simulink model "C_PTES_sim_v2"  (R2025a)
settings: Solver=ode23tb  StartTime=0.0  StopTime=600
PreLoadFcn:
  | Load_Maps
InitFcn:
  | A_init_compressor
StopFcn:
  | % AB_plotHX
  | % AB_plotmap
model workspace (MAT data in the model file):
  Step_time = 1000
  step_time = 200
values from neighbouring files (symbols this model uses):
  DeltaW = 0    [A_init_compressor.m]    (also in B_init_compressor.m = input('Power change: '))
  Ki_tau = 23.1297    [A_init_compressor.m]    (also in B_init_compressor.m = 0.1)
  Kp_tau = 289.6844    [A_init_compressor.m]    (also in B_init_compressor.m = 1)
  omega_step = 376    [A_init_compressor.m]
  stepping_time = 100000    [A_init_compressor.m]    (also in B_init_compressor.m = input('Step time:'))
  tchange = 100000    [A_init_compressor.m]
undefined symbols (not defined in the file or in its folder): z_Qlty_CO2
libraries: simulink_extras x17, slpidlib x9
(part 3 of 3)

== matlab function C_PTES_sim_v2/Cold_side_HXER/Average Temperature ==
  data: u input; y output
function y = fcn(u)

n=length(u)/2;

T_CO2= u(1:n);

y = mean(T_CO2);

== matlab function C_PTES_sim_v2/Hot_side_HXER/Average Temperature1 ==
  data: u input; y1 output; y2 output
function [y1,y2] = fcn(u)

y1 = u(1:end-1);

y2 = u(end);
